simulink model "TiltCopter_TOSTO_v2"  (R2015a)
settings: Solver=ode45  StartTime=0.0  StopTime=10  RelTol=1e-3
values from neighbouring files (symbols this model uses):
  Fx = 0    [Main_tiltCopter_TOSTO.m]    (also in Main_tiltCopter_TOSTO_v2.m)
  Fy = 0    [Main_tiltCopter_TOSTO.m]    (also in Main_tiltCopter_TOSTO_v2.m = 0.2)
  U = [-1; 0; 0; 0]    [Main_tiltCopter_TOSTO.m]    (also in Main_tiltCopter_TOSTO_v2.m = [-1; 0; 0;0])
undefined symbols (not defined in the file or in its folder): b, B0, B1, B2, B3, degtorad, dLMN, g, I_Pi, In, InInv, KaD, KaI, KaN, KaP, Kba, Kbp, Kbq, Kbr, Kdp, Kdq, Kdr, Kip, Kiq, Kir, KPD, KPI, KPP, Kpp, Kpq, Kpr, Kq, KRD, KRI, KRP, Kt, m, m_servo, Mb, MbInv, N, omega_hover, pitchMax, q_servo, rollMax, satp, satq, satr, ServoMotor_Gain, tau, x1, yawRateMax
libraries: aerolibutil x10, simulink x6
(part 1 of 2)
settings Model: PauseTimes=2  Creator=Claudio  LastModifiedBy=Claudio

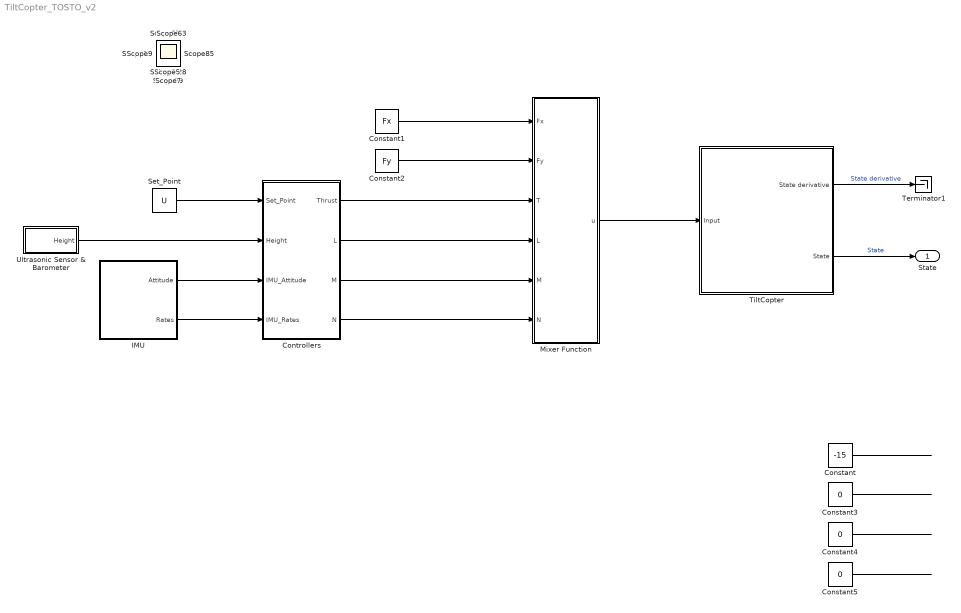
== system TiltCopter_TOSTO_v2 ==
  Constant : Constant  Value=-15
  Constant1 : Constant  Value=Fx
  Constant2 : Constant  Value=Fy
  Constant3 : Constant  Value=0
  Constant4 : Constant  Value=0
  Constant5 : Constant  Value=0
  Controllers : Subsystem
  IMU : Subsystem
  Mixer Function : Subsystem
  Set_Point : Constant  Value=U
  Terminator1 : Terminator
  TiltCopter : Subsystem
      mask Display:
      | % image(imread(''))
      | port_label('input',1,'u')
      | port_label('output',1,'Xdot')
      | port_label('output',2,'X')
  Ultrasonic Sensor & Barometer : Subsystem
  State : Outport
  Scope{,1..29} (30 alike) : Scope
      Scope settings: SaveName=ScopeData2
      Scope1 settings: SaveName=ScopeData3
      Scope10 settings: SaveName=ScopeData14
      Scope11 settings: SaveName=ScopeData15
      Scope12 settings: SaveName=ScopeData16
      Scope13 settings: SaveName=ScopeData17
      Scope14 settings: SaveName=ScopeData18
      Scope15 settings: SaveName=ScopeData19
      Scope16 settings: SaveName=ScopeData20
      Scope17 settings: SaveName=ScopeData21
      Scope18 settings: SaveName=ScopeData22
      Scope19 settings: SaveName=ScopeData23
      Scope2 settings: SaveName=ScopeData4
      Scope20 settings: SaveName=ScopeData24
      Scope21 settings: SaveName=ScopeData25
      Scope22 settings: SaveName=ScopeData26
      Scope23 settings: SaveName=ScopeData27
      Scope24 settings: SaveName=ScopeData28
      Scope25 settings: SaveName=ScopeData31
      Scope26 settings: SaveName=ScopeData30
      Scope27 settings: ShowLegends=on  SaveName=ScopeData32
      Scope28 settings: SaveName=ScopeData33
      Scope29 settings: SaveName=ScopeData34
      Scope3 settings: SaveName=ScopeData5
      Scope4 settings: SaveName=ScopeData8
      Scope5 settings: TimeRange=20  SaveName=ScopeData9
      Scope6 settings: SaveName=ScopeData10
      Scope7 settings: SaveName=ScopeData11
      Scope8 settings: SaveName=ScopeData12
      Scope9 settings: SaveName=ScopeData13
  wires:
  TiltCopter/2(State) -> State/1  "State"
  TiltCopter/1(State derivative) -> Terminator1/1  "State derivative"
  Constant1/1 -> Mixer Function/1(Fx)
  Constant2/1 -> Mixer Function/2(Fy)
  Mixer Function/1(u) -> TiltCopter/1(Input)
  Set_Point/1 -> Controllers/1(Set_Point)
  IMU/1(Attitude) -> Controllers/3(IMU_Attitude)
  IMU/2(Rates) -> Controllers/4(IMU_Rates)
  Ultrasonic Sensor & Barometer/1(Height) -> Controllers/2(Height)
  Constant/1 -> ?
  Constant5/1 -> ?
  Constant4/1 -> ?
  Constant3/1 -> ?
  Controllers/1(Thrust) -> Mixer Function/3(T)
  Controllers/2(L) -> Mixer Function/4(L)
  Controllers/3(M) -> Mixer Function/5(M)
  Controllers/4(N) -> Mixer Function/6(N)

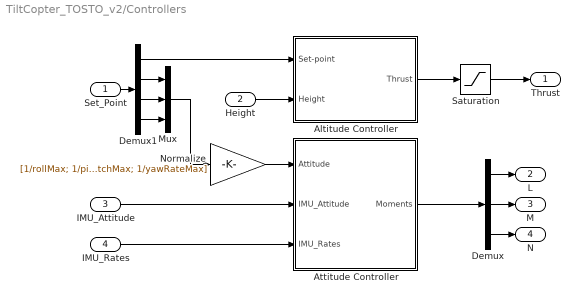
== system TiltCopter_TOSTO_v2/Controllers ==
  Set_Point : Inport
  Height : Inport  Port=2
  IMU_Attitude : Inport  Port=3
  IMU_Rates : Inport  Port=4
  Altitude Controller : Subsystem
  Attitude Controller : Subsystem
  Demux : Demux  Outputs=3
  Demux1 : Demux
  Mux : Mux  Inputs=3
  Normalize : Gain  Gain=[1/rollMax; 1/pitchMax; 1/yawRateMax]
  Saturation : Saturate  UpperLimit=0  LowerLimit=-80
  Thrust : Outport
  L : Outport  Port=2
  M : Outport  Port=3
  N : Outport  Port=4
  wires:
  IMU_Rates/1 -> Attitude Controller/3(IMU_Rates)
  Demux/1 -> L/1
  Demux/2 -> M/1
  Demux/3 -> N/1
  Set_Point/1 -> Demux1/1
  Demux1/3 -> Mux/2
  Demux1/4 -> Mux/3
  IMU_Attitude/1 -> Attitude Controller/2(IMU_Attitude)
  Mux/1 -> Normalize/1
  Normalize/1 -> Attitude Controller/1(Attitude)
  Demux1/1 -> Altitude Controller/1(Set-point)
  Height/1 -> Altitude Controller/2(Height)
  Altitude Controller/1(Thrust) -> Saturation/1
  Saturation/1 -> Thrust/1
  Attitude Controller/1(Moments) -> Demux/1
  Demux1/2 -> Mux/1

== system TiltCopter_TOSTO_v2/IMU ==
  Attitude : Outport
  Rates : Outport  Port=2
  wires:
  [Omega_b] -> Rates/1
  [Alpha_e] -> Attitude/1

== system TiltCopter_TOSTO_v2/Mixer Function ==
  Fx : Inport
  Fy : Inport  Port=2
  T : Inport  Port=3
  L : Inport  Port=4
  M : Inport  Port=5
  N : Inport  Port=6
  Mux1 : Mux
  Mux2 : Mux  Inputs=5
  NONLINEAR mixer : Subsystem
  To Workspace : ToWorkspace  VariableName=Uscita_quad  SaveFormat=Timeseries  SampleTime=-1
  u : Outport
  wires:
  Mux2/1 -> To Workspace/1, u/1
  Fy/1 -> NONLINEAR mixer/2(Fy)
  Fx/1 -> NONLINEAR mixer/1(Fx)
  T/1 -> NONLINEAR mixer/3(T)
  L/1 -> NONLINEAR mixer/4(L)
  N/1 -> NONLINEAR mixer/6(N)
  M/1 -> NONLINEAR mixer/5(M)
  Mux1/1 -> Mux2/5
  NONLINEAR mixer/5(Pulse 1 [ms]) -> Mux1/1
  NONLINEAR mixer/6(Pulse 2 [ms]) -> Mux1/2
  NONLINEAR mixer/7(Pulse 3 [ms]) -> Mux1/3
  NONLINEAR mixer/8(Pulse 4 [ms]) -> Mux1/4
  NONLINEAR mixer/4(Th4 [%]) -> Mux2/4
  NONLINEAR mixer/3(Th3 [%]) -> Mux2/3
  NONLINEAR mixer/2(Th2 [%]) -> Mux2/2
  NONLINEAR mixer/1(Th1 [%]) -> Mux2/1

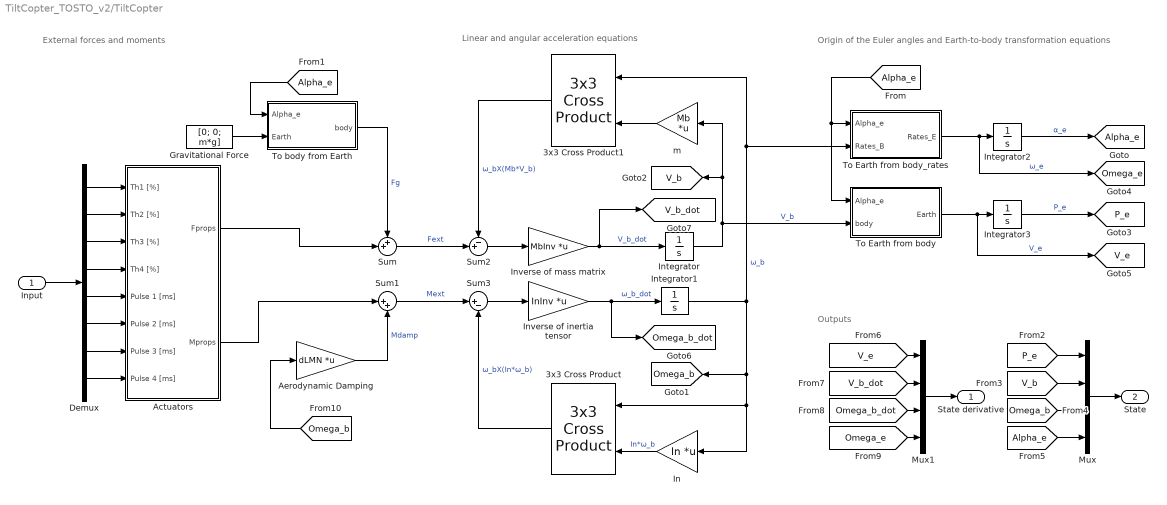
== system TiltCopter_TOSTO_v2/TiltCopter ==
  note: External forces and moments
  note: Outputs
  note: Origin of the Euler angles and Earth-to-body transformation equations
  note: Linear and angular acceleration equations
  Input : Inport
  3x3 Cross Product : aerolibutil/3x3 Cross Product
  3x3 Cross Product1 : aerolibutil/3x3 Cross Product
  Actuators : Subsystem
  Aerodynamic Damping : Gain  Gain=dLMN  Multiplication=Matrix(K*u)
  Demux : Demux  Outputs=8
  Gravitational Force : Constant  Value=[0; 0; m*g]
  In : Gain  Gain=In  Multiplication=Matrix(K*u)
  Integrator : Integrator  InitialCondition=[0; 0; 0]  UpperSaturationLimit=20
  Integrator1 : Integrator  InitialCondition=[0; 0; 0]
  Integrator2 : Integrator  InitialCondition=[0; 0; 0]
  Integrator3 : Integrator  InitialCondition=[0; 0; 0]
  Inverse of inertia tensor : Gain  Gain=InInv  Multiplication=Matrix(K*u)
  Inverse of mass matrix : Gain  Gain=MbInv  Multiplication=Matrix(K*u)
  Mux : Mux
  Mux1 : Mux
  Sum : Sum  Inputs=++|
  Sum1 : Sum  Inputs=|++
  Sum2 : Sum  Inputs=-+|
  Sum3 : Sum  Inputs=|+-
  To Earth from body : MATLAB Function  TreatAsAtomicUnit=on
  To Earth from body_rates : MATLAB Function  TreatAsAtomicUnit=on
  To body from Earth : MATLAB Function  TreatAsAtomicUnit=on
  m : Gain  Gain=Mb  Multiplication=Matrix(K*u)
  State derivative : Outport
  State : Outport  Port=2
  tag scope: Alpha_e=global, Omega_b=global, Omega_b_dot=global, Omega_e=global, P_e=global, V_b=global, V_b_dot=global, V_e=global
  wires:
  To Earth from body_rates/1(Rates_E) -> Integrator2/1, [Omega_e]  "ω_e"
  [P_e] -> Mux/1
  3x3 Cross Product/1 -> Sum3/2  "ω_bX(In*ω_b)"
  [V_b_dot] -> Mux1/2
  Mux/1 -> State/1
  Mux1/1 -> State derivative/1
  [V_b] -> Mux/2
  [Alpha_e] -> Mux/4
  [Omega_b] -> Mux/3
  Demux/4 -> Actuators/4(Th4 [%])
  [Omega_e] -> Mux1/4
  [Omega_b_dot] -> Mux1/3
  [V_e] -> Mux1/1
  Demux/3 -> Actuators/3(Th3 [%])
  Inverse of mass matrix/1 -> Integrator/1, [V_b_dot]  "V_b_dot"
  Integrator/1 -> To Earth from body/2(body), m/1, [V_b]  "V_b"
  [Alpha_e] -> To Earth from body/1(Alpha_e), To Earth from body_rates/1(Alpha_e)
  Integrator1/1 -> To Earth from body_rates/2(Rates_B), 3x3 Cross Product1/1, 3x3 Cross Product/1, In/1, [Omega_b]  "ω_b"
  Sum3/1 -> Inverse of inertia tensor/1
  Sum2/1 -> Inverse of mass matrix/1
  m/1 -> 3x3 Cross Product1/2
  Sum/1 -> Sum2/2  "Fext"
  Sum1/1 -> Sum3/1  "Mext"
  Demux/1 -> Actuators/1(Th1 [%])
  Demux/2 -> Actuators/2(Th2 [%])
  Inverse of inertia tensor/1 -> Integrator1/1, [Omega_b_dot]  "ω_b_dot"
  3x3 Cross Product1/1 -> Sum2/1  "ω_bX(Mb*V_b)"
  Integrator2/1 -> [Alpha_e]  "α_e"
  Aerodynamic Damping/1 -> Sum1/2  "Mdamp"
  Integrator3/1 -> [P_e]  "P_e"
  In/1 -> 3x3 Cross Product/2  "In*ω_b"
  [Omega_b] -> Aerodynamic Damping/1
  To Earth from body/1(Earth) -> [V_e], Integrator3/1  "V_e"
  To body from Earth/1(body) -> Sum/1  "Fg"
  Gravitational Force/1 -> To body from Earth/2(Earth)
  [Alpha_e] -> To body from Earth/1(Alpha_e)
  Input/1 -> Demux/1
  Demux/5 -> Actuators/5(Pulse 1 [ms])
  Demux/6 -> Actuators/6(Pulse 2 [ms])
  Demux/7 -> Actuators/7(Pulse 3 [ms])
  Demux/8 -> Actuators/8(Pulse 4 [ms])
  Actuators/1(Fprops) -> Sum/2
  Actuators/2(Mprops) -> Sum1/1

== system TiltCopter_TOSTO_v2/Ultrasonic Sensor & Barometer ==
  Bias_u : Bias
  Demux : Demux  Outputs=3
  Sum : Sum  Inputs=|++
  Terminator1 : Terminator
  Terminator2 : Terminator
  White Noise_u : RandomNumber  DisableCoverage=on  Variance=0*0.00001  SampleTime=0.01
  Height : Outport
  wires:
  Sum/1 -> Height/1
  Demux/2 -> Terminator1/1  "E"
  [P_e] -> Demux/1
  Bias_u/1 -> Sum/1
  White Noise_u/1 -> Sum/2
  Demux/3 -> Bias_u/1  "D"
  Demux/1 -> Terminator2/1  "N"

== system TiltCopter_TOSTO_v2/Controllers/Altitude Controller ==
  Set-point : Inport
  Height : Inport  Port=2
  Constant : Constant  Value=m*g
  Normalize : Gain
  PD Controller : simulink/Continuous/PID Controller  Controller=PID  TimeDomain=Continuous-time  SampleTime=-1  IntegratorMethod=Forward Euler  FilterMethod=Trapezoidal  Form=Parallel  UseFilter=on  ControllerParametersSource=internal  P=KaP  I=KaI  D=KaD  N=KaN  InitialConditionSource=internal  InitialConditionForIntegrator=0  InitialConditionForFilter=0  ExternalReset=none  LimitOutput=on  UpperSaturationLimit=10  LowerSaturationLimit=-10  LinearizeAsGain=on  AntiWindupMode=back-calculation  Kb=Kba  TrackingMode=off  Kt=1  PParamMin=[]  PParamMax=[]  IParamMin=[]  IParamMax=[]  DParamMin=[]  DParamMax=[]  NParamMin=[]  NParamMax=[]  KbParamMin=[]  KbParamMax=[]  KtParamMin=[]  KtParamMax=[]  POutMin=[]  POutMax=[]  IOutMin=[]  IOutMax=[]  DOutMin=[]  DOutMax=[]  NOutMin=[]  NOutMax=[]  KbOutMin=[]  KbOutMax=[]  KtOutMin=[]  KtOutMax=[]  IntegratorOutMin=[]  IntegratorOutMax=[]  FilterOutMin=[]  FilterOutMax=[]  SumOutMin=[]  SumOutMax=[]  SumI1OutMin=[]  SumI1OutMax=[]  SumI2OutMin=[]  SumI2OutMax=[]  SumI3OutMin=[]  SumI3OutMax=[]  SumDOutMin=[]  SumDOutMax=[]  SaturationOutMin=[]  SaturationOutMax=[]  IntegratorContinuousStateAttributes=''  IntegratorStateMustResolveToSignalObject=off  IntegratorRTWStateStorageClass=Auto  FilterContinuousStateAttributes=''  FilterStateMustResolveToSignalObject=off  FilterRTWStateStorageClass=Auto  DifferentiatorICPrevScaledInput=0  DifferentiatorOutMin=[]  DifferentiatorOutMax=[]
  Sum1 : Sum  Inputs=-+|
  Sum2 : Sum  Inputs=|+-
  Thrust : Outport
  wires:
  Sum2/1 -> PD Controller/1
  Height/1 -> Sum2/2
  Sum1/1 -> Thrust/1
  Constant/1 -> Sum1/1
  Set-point/1 -> Sum2/1
  PD Controller/1 -> Normalize/1
  Normalize/1 -> Sum1/2

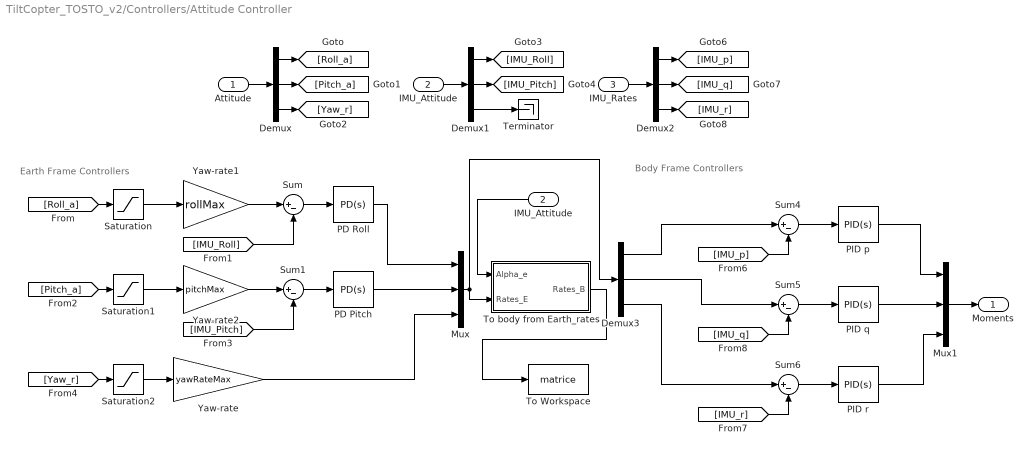
== system TiltCopter_TOSTO_v2/Controllers/Attitude Controller ==
  note: Body Frame Controllers
  note: Earth Frame Controllers
  Attitude : Inport
  IMU_Attitude : Inport  Port=2
  IMU_Rates : Inport  Port=3
  Demux{,1..3} (4 alike) : Demux  Outputs=3
  "IMU_Attitude " : InportShadow  Port=2
  Mux : Mux  Inputs=3
  Mux1 : Mux  Inputs=3
  PD Pitch : simulink/Continuous/PID Controller  Controller=PD  TimeDomain=Continuous-time  SampleTime=-1  IntegratorMethod=Forward Euler  FilterMethod=Forward Euler  Form=Parallel  UseFilter=on  ControllerParametersSource=internal  P=KPP  I=KPI  D=KPD  N=N  InitialConditionSource=internal  InitialConditionForIntegrator=0  InitialConditionForFilter=0  ExternalReset=none  LimitOutput=off  UpperSaturationLimit=inf  LowerSaturationLimit=-inf  LinearizeAsGain=on  AntiWindupMode=none  Kb=1  TrackingMode=off  Kt=1  PParamMin=[]  PParamMax=[]  IParamMin=[]  IParamMax=[]  DParamMin=[]  DParamMax=[]  NParamMin=[]  NParamMax=[]  KbParamMin=[]  KbParamMax=[]  KtParamMin=[]  KtParamMax=[]  POutMin=[]  POutMax=[]  IOutMin=[]  IOutMax=[]  DOutMin=[]  DOutMax=[]  NOutMin=[]  NOutMax=[]  KbOutMin=[]  KbOutMax=[]  KtOutMin=[]  KtOutMax=[]  IntegratorOutMin=[]  IntegratorOutMax=[]  FilterOutMin=[]  FilterOutMax=[]  SumOutMin=[]  SumOutMax=[]  SumI1OutMin=[]  SumI1OutMax=[]  SumI2OutMin=[]  SumI2OutMax=[]  SumI3OutMin=[]  SumI3OutMax=[]  SumDOutMin=[]  SumDOutMax=[]  SaturationOutMin=[]  SaturationOutMax=[]  IntegratorContinuousStateAttributes=''  IntegratorStateMustResolveToSignalObject=off  IntegratorRTWStateStorageClass=Auto  FilterContinuousStateAttributes=''  FilterStateMustResolveToSignalObject=off  FilterRTWStateStorageClass=Auto  DifferentiatorICPrevScaledInput=0  DifferentiatorOutMin=[]  DifferentiatorOutMax=[]
  PD Roll : simulink/Continuous/PID Controller  Controller=PD  TimeDomain=Continuous-time  SampleTime=-1  IntegratorMethod=Forward Euler  FilterMethod=Forward Euler  Form=Parallel  UseFilter=on  ControllerParametersSource=internal  P=KRP  I=KRI  D=KRD  N=N  InitialConditionSource=internal  InitialConditionForIntegrator=0  InitialConditionForFilter=0  ExternalReset=none  LimitOutput=off  UpperSaturationLimit=inf  LowerSaturationLimit=-inf  LinearizeAsGain=on  AntiWindupMode=none  Kb=1  TrackingMode=off  Kt=1  PParamMin=[]  PParamMax=[]  IParamMin=[]  IParamMax=[]  DParamMin=[]  DParamMax=[]  NParamMin=[]  NParamMax=[]  KbParamMin=[]  KbParamMax=[]  KtParamMin=[]  KtParamMax=[]  POutMin=[]  POutMax=[]  IOutMin=[]  IOutMax=[]  DOutMin=[]  DOutMax=[]  NOutMin=[]  NOutMax=[]  KbOutMin=[]  KbOutMax=[]  KtOutMin=[]  KtOutMax=[]  IntegratorOutMin=[]  IntegratorOutMax=[]  FilterOutMin=[]  FilterOutMax=[]  SumOutMin=[]  SumOutMax=[]  SumI1OutMin=[]  SumI1OutMax=[]  SumI2OutMin=[]  SumI2OutMax=[]  SumI3OutMin=[]  SumI3OutMax=[]  SumDOutMin=[]  SumDOutMax=[]  SaturationOutMin=[]  SaturationOutMax=[]  IntegratorContinuousStateAttributes=''  IntegratorStateMustResolveToSignalObject=off  IntegratorRTWStateStorageClass=Auto  FilterContinuousStateAttributes=''  FilterStateMustResolveToSignalObject=off  FilterRTWStateStorageClass=Auto  DifferentiatorICPrevScaledInput=0  DifferentiatorOutMin=[]  DifferentiatorOutMax=[]
  PID p : simulink/Continuous/PID Controller  Controller=PID  TimeDomain=Continuous-time  SampleTime=-1  IntegratorMethod=Forward Euler  FilterMethod=Forward Euler  Form=Parallel  UseFilter=on  ControllerParametersSource=internal  P=Kpp  I=Kip  D=Kdp  N=N  InitialConditionSource=internal  InitialConditionForIntegrator=0  InitialConditionForFilter=0  ExternalReset=none  LimitOutput=on  UpperSaturationLimit=satp  LowerSaturationLimit=-satp  LinearizeAsGain=on  AntiWindupMode=back-calculation  Kb=Kbp  TrackingMode=off  Kt=1  PParamMin=[]  PParamMax=[]  IParamMin=[]  IParamMax=[]  DParamMin=[]  DParamMax=[]  NParamMin=[]  NParamMax=[]  KbParamMin=[]  KbParamMax=[]  KtParamMin=[]  KtParamMax=[]  POutMin=[]  POutMax=[]  IOutMin=[]  IOutMax=[]  DOutMin=[]  DOutMax=[]  NOutMin=[]  NOutMax=[]  KbOutMin=[]  KbOutMax=[]  KtOutMin=[]  KtOutMax=[]  IntegratorOutMin=[]  IntegratorOutMax=[]  FilterOutMin=[]  FilterOutMax=[]  SumOutMin=[]  SumOutMax=[]  SumI1OutMin=[]  SumI1OutMax=[]  SumI2OutMin=[]  SumI2OutMax=[]  SumI3OutMin=[]  SumI3OutMax=[]  SumDOutMin=[]  SumDOutMax=[]  SaturationOutMin=[]  SaturationOutMax=[]  IntegratorContinuousStateAttributes=''  IntegratorStateMustResolveToSignalObject=off  IntegratorRTWStateStorageClass=Auto  FilterContinuousStateAttributes=''  FilterStateMustResolveToSignalObject=off  FilterRTWStateStorageClass=Auto  DifferentiatorICPrevScaledInput=0  DifferentiatorOutMin=[]  DifferentiatorOutMax=[]
  PID q : simulink/Continuous/PID Controller  Controller=PID  TimeDomain=Continuous-time  SampleTime=-1  IntegratorMethod=Forward Euler  FilterMethod=Forward Euler  Form=Parallel  UseFilter=on  ControllerParametersSource=internal  P=Kpq  I=Kiq  D=Kdq  N=N  InitialConditionSource=internal  InitialConditionForIntegrator=0  InitialConditionForFilter=0  ExternalReset=none  LimitOutput=on  UpperSaturationLimit=satq  LowerSaturationLimit=-satq  LinearizeAsGain=on  AntiWindupMode=back-calculation  Kb=Kbq  TrackingMode=off  Kt=1  PParamMin=[]  PParamMax=[]  IParamMin=[]  IParamMax=[]  DParamMin=[]  DParamMax=[]  NParamMin=[]  NParamMax=[]  KbParamMin=[]  KbParamMax=[]  KtParamMin=[]  KtParamMax=[]  POutMin=[]  POutMax=[]  IOutMin=[]  IOutMax=[]  DOutMin=[]  DOutMax=[]  NOutMin=[]  NOutMax=[]  KbOutMin=[]  KbOutMax=[]  KtOutMin=[]  KtOutMax=[]  IntegratorOutMin=[]  IntegratorOutMax=[]  FilterOutMin=[]  FilterOutMax=[]  SumOutMin=[]  SumOutMax=[]  SumI1OutMin=[]  SumI1OutMax=[]  SumI2OutMin=[]  SumI2OutMax=[]  SumI3OutMin=[]  SumI3OutMax=[]  SumDOutMin=[]  SumDOutMax=[]  SaturationOutMin=[]  SaturationOutMax=[]  IntegratorContinuousStateAttributes=''  IntegratorStateMustResolveToSignalObject=off  IntegratorRTWStateStorageClass=Auto  FilterContinuousStateAttributes=''  FilterStateMustResolveToSignalObject=off  FilterRTWStateStorageClass=Auto  DifferentiatorICPrevScaledInput=0  DifferentiatorOutMin=[]  DifferentiatorOutMax=[]
  PID r : simulink/Continuous/PID Controller  Controller=PID  TimeDomain=Continuous-time  SampleTime=-1  IntegratorMethod=Forward Euler  FilterMethod=Forward Euler  Form=Parallel  UseFilter=on  ControllerParametersSource=internal  P=Kpr  I=Kir  D=Kdr  N=N  InitialConditionSource=internal  InitialConditionForIntegrator=0  InitialConditionForFilter=0  ExternalReset=none  LimitOutput=on  UpperSaturationLimit=satr  LowerSaturationLimit=-satr  LinearizeAsGain=on  AntiWindupMode=back-calculation  Kb=Kbr  TrackingMode=off  Kt=1  PParamMin=[]  PParamMax=[]  IParamMin=[]  IParamMax=[]  DParamMin=[]  DParamMax=[]  NParamMin=[]  NParamMax=[]  KbParamMin=[]  KbParamMax=[]  KtParamMin=[]  KtParamMax=[]  POutMin=[]  POutMax=[]  IOutMin=[]  IOutMax=[]  DOutMin=[]  DOutMax=[]  NOutMin=[]  NOutMax=[]  KbOutMin=[]  KbOutMax=[]  KtOutMin=[]  KtOutMax=[]  IntegratorOutMin=[]  IntegratorOutMax=[]  FilterOutMin=[]  FilterOutMax=[]  SumOutMin=[]  SumOutMax=[]  SumI1OutMin=[]  SumI1OutMax=[]  SumI2OutMin=[]  SumI2OutMax=[]  SumI3OutMin=[]  SumI3OutMax=[]  SumDOutMin=[]  SumDOutMax=[]  SaturationOutMin=[]  SaturationOutMax=[]  IntegratorContinuousStateAttributes=''  IntegratorStateMustResolveToSignalObject=off  IntegratorRTWStateStorageClass=Auto  FilterContinuousStateAttributes=''  FilterStateMustResolveToSignalObject=off  FilterRTWStateStorageClass=Auto  DifferentiatorICPrevScaledInput=0  DifferentiatorOutMin=[]  DifferentiatorOutMax=[]
  Saturation : Saturate  UpperLimit=1  LowerLimit=-1
  Saturation1 : Saturate  UpperLimit=1  LowerLimit=-1
  Saturation2 : Saturate  UpperLimit=1  LowerLimit=-1
  Sum{,1,4..6} (5 alike) : Sum  Inputs=|+-
  Terminator : Terminator
  To Workspace : ToWorkspace  VariableName=matrice  SaveFormat=Timeseries  SampleTime=-1
  To body from Earth_rates : MATLAB Function  TreatAsAtomicUnit=on
  Yaw-rate : Gain  Gain=yawRateMax
  Yaw-rate1 : Gain  Gain=rollMax
  Yaw-rate2 : Gain  Gain=pitchMax
  Moments : Outport
  wires:
  Sum4/1 -> PID p/1
  IMU_Attitude/1 -> Demux1/1
  Attitude/1 -> Demux/1
  Demux/3 -> [Yaw_r]
  IMU_Rates/1 -> Demux2/1
  [IMU_Pitch] -> Sum1/2
  [Pitch_a] -> Saturation1/1
  [IMU_Roll] -> Sum/2
  [Roll_a] -> Saturation/1
  Mux1/1 -> Moments/1
  PD Roll/1 -> Mux/1
  [Yaw_r] -> Saturation2/1
  PD Pitch/1 -> Mux/2
  Sum5/1 -> PID q/1
  PID r/1 -> Mux1/3
  PID p/1 -> Mux1/1
  Sum6/1 -> PID r/1
  PID q/1 -> Mux1/2
  Demux/2 -> [Pitch_a]
  Demux2/3 -> [IMU_r]
  Demux1/1 -> [IMU_Roll]
  Demux/1 -> [Roll_a]
  Demux2/1 -> [IMU_p]
  Demux1/3 -> Terminator/1
  Demux2/2 -> [IMU_q]
  Demux1/2 -> [IMU_Pitch]
  Sum/1 -> PD Roll/1
  Sum1/1 -> PD Pitch/1
  Saturation1/1 -> Yaw-rate2/1
  Yaw-rate1/1 -> Sum/1
  Yaw-rate2/1 -> Sum1/1
  Demux3/1 -> Sum4/1
  [IMU_p] -> Sum4/2
  Demux3/2 -> Sum5/1
  Demux3/3 -> Sum6/1
  [IMU_q] -> Sum5/2
  [IMU_r] -> Sum6/2
  Yaw-rate/1 -> Mux/3
  Saturation/1 -> Yaw-rate1/1
  Saturation2/1 -> Yaw-rate/1
  "IMU_Attitude "/1 -> To body from Earth_rates/1(Alpha_e)
  To body from Earth_rates/1(Rates_B) -> To Workspace/1
  Mux/1 -> Demux3/1, To body from Earth_rates/2(Rates_E)

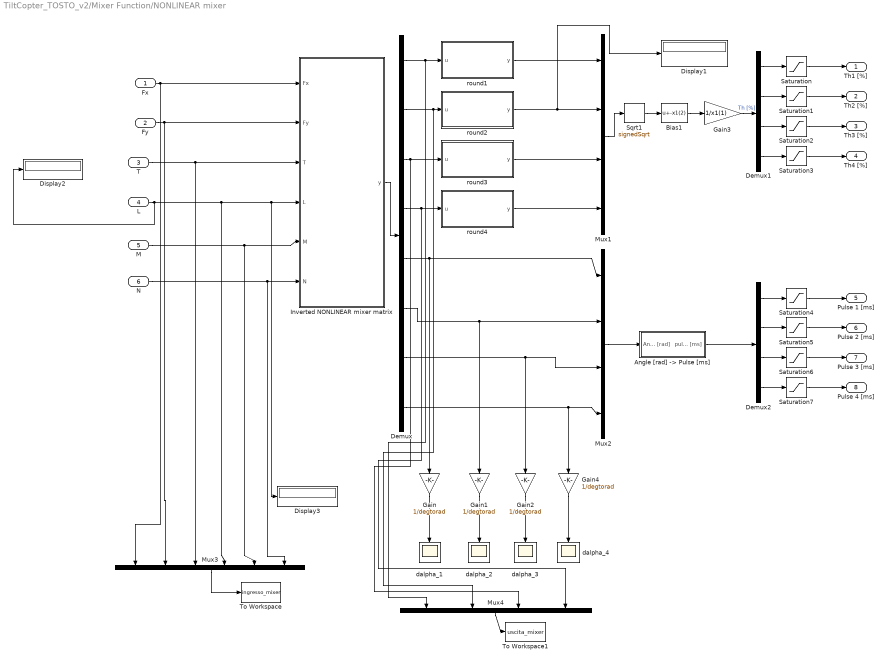
== system TiltCopter_TOSTO_v2/Mixer Function/NONLINEAR mixer ==
  Fx : Inport
  Fy : Inport  Port=2
  T : Inport  Port=3
  L : Inport  Port=4
  M : Inport  Port=5
  N : Inport  Port=6
  "Angle [rad] -> Pulse [ms]" : Subsystem
  Bias1 : Bias  Bias=-x1(2)
  Demux : Demux  Outputs=8
  Demux1 : Demux
  Demux2 : Demux
  Display1 : Display
  Display2 : Display
  Display3 : Display
  Gain{,1..2,4} (4 alike) : Gain  Gain=1/degtorad
  Gain3 : Gain  Gain=1/x1(1)
  Inverted NONLINEAR mixer matrix : MATLAB Function  TreatAsAtomicUnit=on
  Mux1 : Mux
  Mux2 : Mux
  Mux3 : Mux  Inputs=6
  Mux4 : Mux
  Saturation{,1..3} (4 alike) : Saturate  UpperLimit=100  LowerLimit=0
  Saturation{4..7} (4 alike) : Saturate  UpperLimit=2000  LowerLimit=1000
  Sqrt1 : Sqrt  Operator=signedSqrt  SaturateOnIntegerOverflow=on
  To Workspace : ToWorkspace  VariableName=ingresso_mixer  SaveFormat=Structure With Time  SampleTime=-1
  To Workspace1 : ToWorkspace  VariableName=uscita_mixer  SaveFormat=Structure With Time  SampleTime=-1
  dalpha_{1..4} (4 alike) : Scope
      dalpha_3 settings: SaveName=ScopeData6
      dalpha_4 settings: SaveName=ScopeData7
  round1 : MATLAB Function  TreatAsAtomicUnit=on
  round2 : MATLAB Function  TreatAsAtomicUnit=on
  round3 : MATLAB Function  TreatAsAtomicUnit=on
  round4 : MATLAB Function  TreatAsAtomicUnit=on
  Th1 [%] : Outport
  Th2 [%] : Outport  Port=2
  Th3 [%] : Outport  Port=3
  Th4 [%] : Outport  Port=4
  Pulse 1 [ms] : Outport  Port=5
  Pulse 2 [ms] : Outport  Port=6
  Pulse 3 [ms] : Outport  Port=7
  Pulse 4 [ms] : Outport  Port=8
  wires:
  round1/1(y) -> Mux1/1
  Saturation6/1 -> Pulse 3 [ms]/1
  Demux2/1 -> Saturation4/1
  Demux2/3 -> Saturation6/1
  Demux/4 -> Mux4/4, round4/1(u)
  Saturation2/1 -> Th3 [%]/1
  Demux1/2 -> Saturation1/1
  Demux1/1 -> Saturation/1
  Demux1/3 -> Saturation2/1
  Demux1/4 -> Saturation3/1
  Saturation1/1 -> Th2 [%]/1
  Gain3/1 -> Demux1/1  "Th [%]"
  Sqrt1/1 -> Bias1/1
  Mux1/1 -> Sqrt1/1
  Demux/1 -> Mux4/1, round1/1(u)
  Bias1/1 -> Gain3/1
  Saturation3/1 -> Th4 [%]/1
  Saturation/1 -> Th1 [%]/1
  Demux2/2 -> Saturation5/1
  round2/1(y) -> Display1/1, Mux1/2
  round4/1(y) -> Mux1/4
  Demux/7 -> Gain2/1, Mux2/3
  Demux/5 -> Gain/1, Mux2/1
  Demux/6 -> Mux2/2, Gain1/1
  Mux2/1 -> "Angle [rad] -> Pulse [ms]"/1(Angle [rad])
  Demux2/4 -> Saturation7/1
  Demux/3 -> round3/1(u), Mux4/3
  Demux/8 -> Mux2/4, Gain4/1
  "Angle [rad] -> Pulse [ms]"/1(pulse [ms]) -> Demux2/1
  Saturation4/1 -> Pulse 1 [ms]/1
  Saturation5/1 -> Pulse 2 [ms]/1
  Saturation7/1 -> Pulse 4 [ms]/1
  Gain1/1 -> dalpha_2/1
  Gain/1 -> dalpha_1/1
  Gain2/1 -> dalpha_3/1
  Gain4/1 -> dalpha_4/1
  round3/1(y) -> Mux1/3
  Inverted NONLINEAR mixer matrix/1(y) -> Demux/1
  Demux/2 -> Mux4/2, round2/1(u)
  Fx/1 -> Mux3/1, Inverted NONLINEAR mixer matrix/1(Fx)
  Fy/1 -> Inverted NONLINEAR mixer matrix/2(Fy), Mux3/2
  T/1 -> Inverted NONLINEAR mixer matrix/3(T), Mux3/3
  L/1 -> Mux3/4, Display3/1, Inverted NONLINEAR mixer matrix/4(L), Display2/1
  M/1 -> Mux3/5, Inverted NONLINEAR mixer matrix/5(M)
  N/1 -> Mux3/6, Inverted NONLINEAR mixer matrix/6(N)
  Mux3/1 -> To Workspace/1
  Mux4/1 -> To Workspace1/1

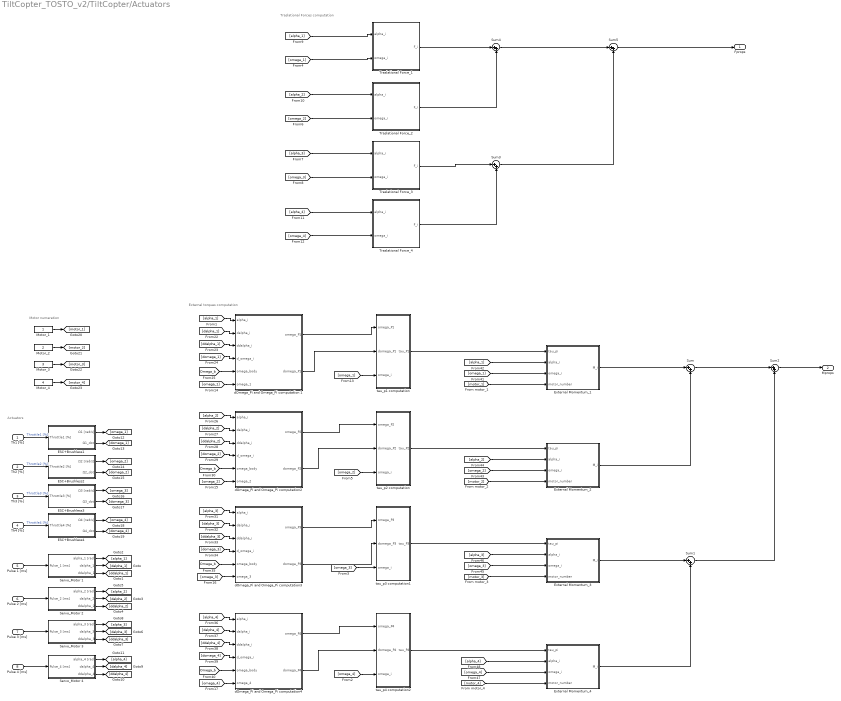
== system TiltCopter_TOSTO_v2/TiltCopter/Actuators ==
  note: Actuators
  note: Motor numeration
  note: External torques computation
  note: Traslational Forces computation
  Th1 [%] : Inport
  Th2 [%] : Inport  Port=2
  Th3 [%] : Inport  Port=3
  Th4 [%] : Inport  Port=4
  Pulse 1 [ms] : Inport  Port=5
  Pulse 2 [ms] : Inport  Port=6
  Pulse 3 [ms] : Inport  Port=7
  Pulse 4 [ms] : Inport  Port=8
  ESC+Brushless1 : Subsystem
  ESC+Brushless2 : Subsystem
  ESC+Brushless3 : Subsystem
  ESC+Brushless4 : Subsystem
  External Momentum_1 : Subsystem
  External Momentum_2 : Subsystem
  External Momentum_3 : Subsystem
  External Momentum_4 : Subsystem
  Motor_1 : Constant
  Motor_2 : Constant  Value=2
  Motor_3 : Constant  Value=3
  Motor_4 : Constant  Value=4
  Servo_Motor 1 : Subsystem
  Servo_Motor 2 : Subsystem
  Servo_Motor 3 : Subsystem
  Servo_Motor 4 : Subsystem
  Sum{,1..5} (6 alike) : Sum  Inputs=|++
  Traslational Force_1 : Subsystem
  Traslational Force_2 : Subsystem
  Traslational Force_3 : Subsystem
  Traslational Force_4 : Subsystem
  dOmega_Pi and Omega_Pi computation 1 : Subsystem
  dOmega_Pi and Omega_Pi computation2 : Subsystem
  dOmega_Pi and Omega_Pi computation3 : Subsystem
  dOmega_Pi and Omega_Pi computation4 : Subsystem
  tau_p1 computation : Subsystem
  tau_p2 computation : Subsystem
  tau_p3 computation1 : Subsystem
  tau_p4 computation2 : Subsystem
  Fprops : Outport
  Mprops : Outport  Port=2
  wires:
  Th1 [%]/1 -> ESC+Brushless1/1(Throttle1 [%])  "Throttle1 [%]"
  Th2 [%]/1 -> ESC+Brushless2/1(Throttle2 [%])  "Throttle2 [%]"
  Th4 [%]/1 -> ESC+Brushless4/1(Throttle4 [%])  "Throttle4 [%]"
  Th3 [%]/1 -> ESC+Brushless3/1(Throttle3 [%])  "Throttle3 [%]"
  Pulse 1 [ms]/1 -> Servo_Motor 1/1(Pulse_1 [ms])
  Pulse 2 [ms]/1 -> Servo_Motor 2/1(Pulse_2 [ms])
  Pulse 3 [ms]/1 -> Servo_Motor 3/1(Pulse_3 [ms])
  Pulse 4 [ms]/1 -> Servo_Motor 4/1(Pulse_4 [ms])
  Servo_Motor 1/2(dalpha_1) -> [dalpha_1]
  Servo_Motor 1/3(ddalpha_1) -> [ddalpha_1]
  Servo_Motor 3/1(alpha_3 [rad]) -> [alpha_3]
  Servo_Motor 3/3(ddalpha_3) -> [ddalpha_3]
  Servo_Motor 3/2(dalpha_3) -> [dalpha_3]
  Servo_Motor 2/3(ddalpha_2) -> [ddalpha_2]
  Servo_Motor 2/2(dalpha_2) -> [dalpha_2]
  Servo_Motor 2/1(alpha_2 [rad]) -> [alpha_2]
  Servo_Motor 1/1(alpha_1 [rad]) -> [alpha_1]
  Servo_Motor 4/1(alpha_4 [rad]) -> [alpha_4]
  Servo_Motor 4/2(dalpha_4) -> [dalpha_4]
  Servo_Motor 4/3(ddalpha_4) -> [ddalpha_4]
  ESC+Brushless1/1(Ω1 [rad/s]) -> [omega_1]
  ESC+Brushless1/2(Ω1_dot) -> [domega_1]
  ESC+Brushless2/1(Ω2 [rad/s]) -> [omega_2]
  ESC+Brushless2/2(Ω2_dot) -> [domega_2]
  ESC+Brushless3/1(Ω3 [rad/s]) -> [omega_3]
  ESC+Brushless3/2(Ω3_dot) -> [domega_3]
  ESC+Brushless4/1(Ω4 [rad/s]) -> [omega_4]
  ESC+Brushless4/2("Ω4_dot ") -> [domega_4]
  [alpha_1] -> dOmega_Pi and Omega_Pi computation 1/1(alpha_i)
  [dalpha_1] -> dOmega_Pi and Omega_Pi computation 1/2(dalpha_i)
  [ddalpha_1] -> dOmega_Pi and Omega_Pi computation 1/3(ddalpha_i)
  [domega_1] -> dOmega_Pi and Omega_Pi computation 1/4(d_omega_i)
  [Omega_b] -> dOmega_Pi and Omega_Pi computation 1/5(omega_body)
  [alpha_2] -> dOmega_Pi and Omega_Pi computation2/1(alpha_i)
  [dalpha_2] -> dOmega_Pi and Omega_Pi computation2/2(dalpha_i)
  [ddalpha_2] -> dOmega_Pi and Omega_Pi computation2/3(ddalpha_i)
  [domega_2] -> dOmega_Pi and Omega_Pi computation2/4(d_omega_i)
  [Omega_b] -> dOmega_Pi and Omega_Pi computation2/5(omega_body)
  [alpha_3] -> dOmega_Pi and Omega_Pi computation3/1(alpha_i)
  [dalpha_3] -> dOmega_Pi and Omega_Pi computation3/2(dalpha_i)
  [ddalpha_3] -> dOmega_Pi and Omega_Pi computation3/3(ddalpha_i)
  [domega_3] -> dOmega_Pi and Omega_Pi computation3/4(d_omega_i)
  [Omega_b] -> dOmega_Pi and Omega_Pi computation3/5(omega_body)
  [alpha_4] -> dOmega_Pi and Omega_Pi computation4/1(alpha_i)
  [dalpha_4] -> dOmega_Pi and Omega_Pi computation4/2(dalpha_i)
  [ddalpha_4] -> dOmega_Pi and Omega_Pi computation4/3(ddalpha_i)
  [domega_4] -> dOmega_Pi and Omega_Pi computation4/4(d_omega_i)
  [Omega_b] -> dOmega_Pi and Omega_Pi computation4/5(omega_body)
  dOmega_Pi and Omega_Pi computation 1/1(omega_P1) -> tau_p1 computation/1(omega_P1)
  dOmega_Pi and Omega_Pi computation 1/2(domega_P1) -> tau_p1 computation/2(domega_P1)
  dOmega_Pi and Omega_Pi computation2/1(omega_P2) -> tau_p2 computation/1(omega_P2)
  dOmega_Pi and Omega_Pi computation2/2(domega_P2) -> tau_p2 computation/2(domega_P2)
  dOmega_Pi and Omega_Pi computation3/1(omega_P3) -> tau_p3 computation1/1(omega_P3)
  dOmega_Pi and Omega_Pi computation3/2(domega_P3) -> tau_p3 computation1/2(domega_P3)
  dOmega_Pi and Omega_Pi computation4/1(omega_P4) -> tau_p4 computation2/1(omega_P4)
  dOmega_Pi and Omega_Pi computation4/2(domega_P4) -> tau_p4 computation2/2(domega_P4)
  tau_p1 computation/1(tau_P1) -> External Momentum_1/1(tau_pi)
  [alpha_1] -> External Momentum_1/2(alpha_i)
  [omega_1] -> External Momentum_1/3(omega_i)
  tau_p2 computation/1(tau_P2) -> External Momentum_2/1(tau_pi)
  [alpha_2] -> External Momentum_2/2(alpha_i)
  [omega_2] -> External Momentum_2/3(omega_i)
  [motor_2] -> External Momentum_2/4(motor_number)
  tau_p3 computation1/1(tau_P3) -> External Momentum_3/1(tau_pi)
  [alpha_3] -> External Momentum_3/2(alpha_i)
  [omega_3] -> External Momentum_3/3(omega_i)
  [motor_3] -> External Momentum_3/4(motor_number)
  [alpha_4] -> External Momentum_4/2(alpha_i)
  [omega_4] -> External Momentum_4/3(omega_i)
  [motor_4] -> External Momentum_4/4(motor_number)
  tau_p4 computation2/1(tau_P4) -> External Momentum_4/1(tau_pi)
  External Momentum_1/1(M_i) -> Sum/1
  External Momentum_3/1(M_i) -> Sum1/1
  External Momentum_4/1(M_i) -> Sum1/2
  Sum/1 -> Sum2/1
  Sum2/1 -> Mprops/1
  [omega_2] -> Traslational Force_2/2(omega_i)
  [alpha_1] -> Traslational Force_1/1(alpha_i)
  [omega_1] -> Traslational Force_1/2(omega_i)
  [alpha_2] -> Traslational Force_2/1(alpha_i)
  Motor_1/1 -> [motor_1]
  Motor_2/1 -> [motor_2]
  Motor_3/1 -> [motor_3]
  Motor_4/1 -> [motor_4]
  [omega_3] -> Traslational Force_3/2(omega_i)
  [alpha_3] -> Traslational Force_3/1(alpha_i)
  [omega_4] -> Traslational Force_4/2(omega_i)
  [alpha_4] -> Traslational Force_4/1(alpha_i)
  Traslational Force_3/1(F_i) -> Sum3/1
  Traslational Force_4/1(F_i) -> Sum3/2
  Traslational Force_1/1(F_i) -> Sum4/1
  Traslational Force_2/1(F_i) -> Sum4/2
  Sum4/1 -> Sum5/1
  Sum3/1 -> Sum5/2
  Sum5/1 -> Fprops/1
  [omega_4] -> tau_p4 computation2/3(omega_i)
  [omega_3] -> tau_p3 computation1/3(omega_i)
  [omega_2] -> tau_p2 computation/3(omega_i)
  [omega_1] -> tau_p1 computation/3(omega_i)
  Sum1/1 -> Sum2/2
  External Momentum_2/1(M_i) -> Sum/2
  [motor_1] -> External Momentum_1/4(motor_number)
  [omega_1] -> dOmega_Pi and Omega_Pi computation 1/6(omega_1)
  [omega_2] -> dOmega_Pi and Omega_Pi computation2/6(omega_2)
  [omega_3] -> dOmega_Pi and Omega_Pi computation3/6(omega_3)
  [omega_4] -> dOmega_Pi and Omega_Pi computation4/6(omega_4)

== system TiltCopter_TOSTO_v2/Mixer Function/NONLINEAR mixer/Angle [rad] -> Pulse [ms] ==
  Angle [rad] : Inport
  Add : Sum
  Constant : Constant  Value=q_servo
  Linear fitting gain : Gain  Gain=m_servo
  pulse [ms] : Outport
  wires:
  Angle [rad]/1 -> Linear fitting gain/1
  Constant/1 -> Add/2
  Linear fitting gain/1 -> Add/1
  Add/1 -> pulse [ms]/1

== system TiltCopter_TOSTO_v2/TiltCopter/Actuators/ESC+Brushless1 ==
  note: questo blocco è stato introdotto per avere in
      | uscita l'accelerazione e la velocità
  Throttle1 [%] : Inport
  Bias : Bias  Bias=x1(2)
  Derivative : Derivative
  Gain : Gain  Gain=x1(1)
  Transfer Fcn : TransferFcn  Denominator=[(tau) 1]
  Ω1 [rad/s] : Outport
  Ω1_dot : Outport  Port=2
  wires:
  Bias/1 -> Ω1 [rad/s]/1
  Throttle1 [%]/1 -> Transfer Fcn/1
  Transfer Fcn/1 -> Gain/1
  Gain/1 -> Bias/1, Derivative/1
  Derivative/1 -> Ω1_dot/1

== system TiltCopter_TOSTO_v2/TiltCopter/Actuators/ESC+Brushless2 ==
  Throttle2 [%] : Inport
  Bias : Bias  Bias=x1(2)
  Derivative : Derivative
  Gain : Gain  Gain=x1(1)
  Transfer Fcn : TransferFcn  Denominator=[(tau) 1]
  Ω2 [rad/s] : Outport
  Ω2_dot : Outport  Port=2
  wires:
  Bias/1 -> Ω2 [rad/s]/1
  Throttle2 [%]/1 -> Transfer Fcn/1
  Transfer Fcn/1 -> Gain/1
  Gain/1 -> Derivative/1, Bias/1
  Derivative/1 -> Ω2_dot/1

== system TiltCopter_TOSTO_v2/TiltCopter/Actuators/ESC+Brushless3 ==
  Throttle3 [%] : Inport
  Bias : Bias  Bias=x1(2)
  Derivative : Derivative
  Gain : Gain  Gain=x1(1)
  Switch : Switch  Criteria=u2 > Threshold
  Transfer Fcn : TransferFcn  Denominator=[(tau) 1]
  Ω3 [rad/s] : Outport
  Ω3_dot : Outport  Port=2
  wires:
  Gain/1 -> Bias/1
  Bias/1 -> Derivative/1, Ω3 [rad/s]/1
  Throttle3 [%]/1 -> Transfer Fcn/1
  Transfer Fcn/1 -> Gain/1
  Derivative/1 -> Ω3_dot/1

== system TiltCopter_TOSTO_v2/TiltCopter/Actuators/ESC+Brushless4 ==
  Throttle4 [%] : Inport
  Bias : Bias  Bias=x1(2)
  Derivative : Derivative
  Gain : Gain  Gain=x1(1)
  Transfer Fcn : TransferFcn  Denominator=[(tau) 1]
  Ω4 [rad/s] : Outport
  "Ω4_dot " : Outport  Port=2
  wires:
  Gain/1 -> Bias/1
  Throttle4 [%]/1 -> Transfer Fcn/1
  Transfer Fcn/1 -> Gain/1
  Derivative/1 -> "Ω4_dot "/1
  Bias/1 -> Derivative/1, Ω4 [rad/s]/1

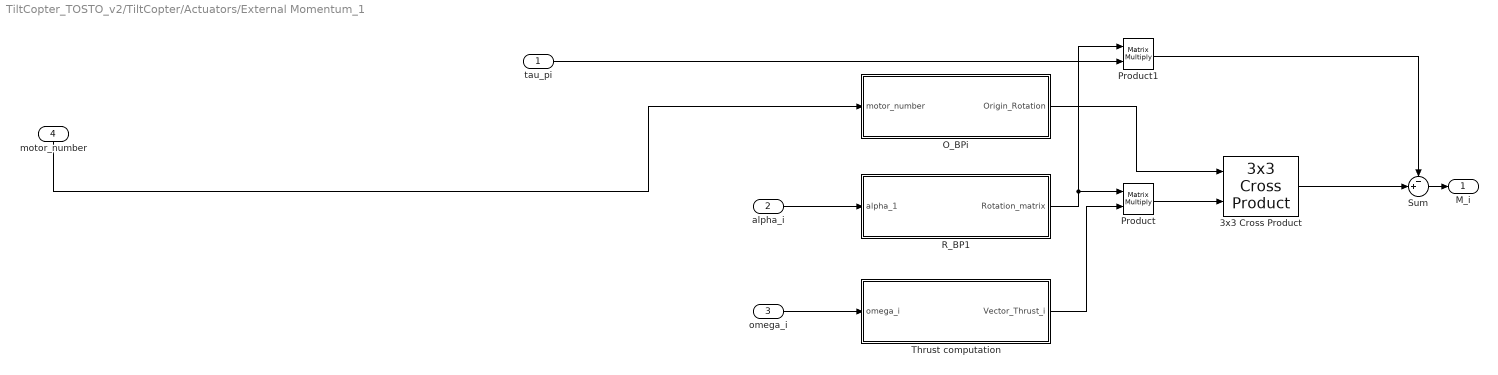
== system TiltCopter_TOSTO_v2/TiltCopter/Actuators/External Momentum_1 ==
  tau_pi : Inport
  alpha_i : Inport  Port=2
  omega_i : Inport  Port=3
  motor_number : Inport  Port=4
  3x3 Cross Product : aerolibutil/3x3 Cross Product
  O_BPi : MATLAB Function  TreatAsAtomicUnit=on
  Product : Product  Multiplication=Matrix(*)
  Product1 : Product  Multiplication=Matrix(*)
  R_BP1 : MATLAB Function  TreatAsAtomicUnit=on
  Sum : Sum  Inputs=-+|
  Thrust computation : Subsystem
  M_i : Outport
  wires:
  Sum/1 -> M_i/1
  R_BP1/1(Rotation_matrix) -> Product1/1, Product/1
  alpha_i/1 -> R_BP1/1(alpha_1)
  Product/1 -> 3x3 Cross Product/2
  tau_pi/1 -> Product1/2
  motor_number/1 -> O_BPi/1(motor_number)
  omega_i/1 -> Thrust computation/1(omega_i)
  Thrust computation/1(Vector_Thrust_i) -> Product/2
  3x3 Cross Product/1 -> Sum/2
  Product1/1 -> Sum/1
  O_BPi/1(Origin_Rotation) -> 3x3 Cross Product/1

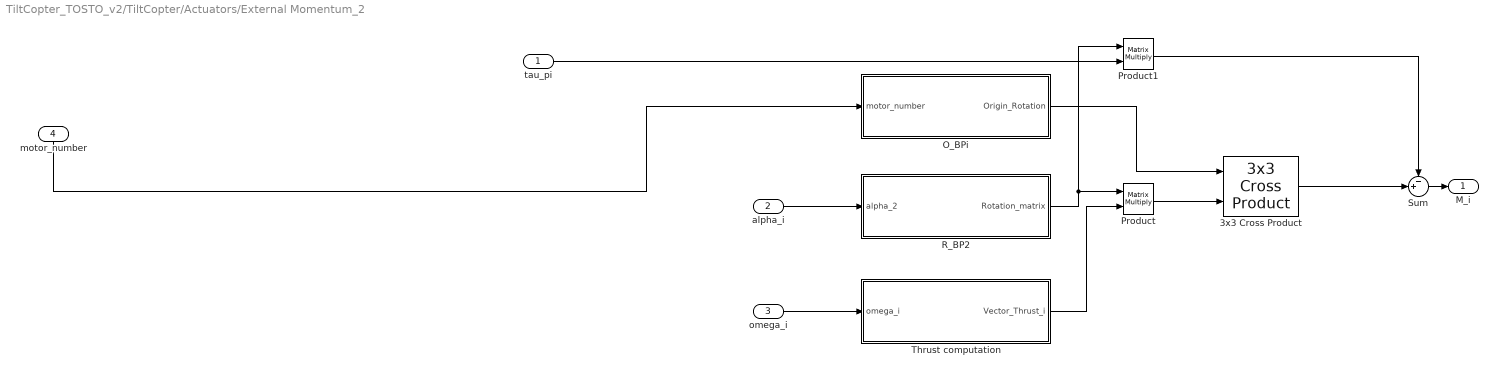
== system TiltCopter_TOSTO_v2/TiltCopter/Actuators/External Momentum_2 ==
  tau_pi : Inport
  alpha_i : Inport  Port=2
  omega_i : Inport  Port=3
  motor_number : Inport  Port=4
  3x3 Cross Product : aerolibutil/3x3 Cross Product
  O_BPi : MATLAB Function  TreatAsAtomicUnit=on
  Product : Product  Multiplication=Matrix(*)
  Product1 : Product  Multiplication=Matrix(*)
  R_BP2 : MATLAB Function  TreatAsAtomicUnit=on
  Sum : Sum  Inputs=-+|
  Thrust computation : Subsystem
  M_i : Outport
  wires:
  Sum/1 -> M_i/1
  R_BP2/1(Rotation_matrix) -> Product1/1, Product/1
  alpha_i/1 -> R_BP2/1(alpha_2)
  Product/1 -> 3x3 Cross Product/2
  tau_pi/1 -> Product1/2
  motor_number/1 -> O_BPi/1(motor_number)
  omega_i/1 -> Thrust computation/1(omega_i)
  Thrust computation/1(Vector_Thrust_i) -> Product/2
  3x3 Cross Product/1 -> Sum/2
  Product1/1 -> Sum/1
  O_BPi/1(Origin_Rotation) -> 3x3 Cross Product/1

== system TiltCopter_TOSTO_v2/TiltCopter/Actuators/External Momentum_3 ==
  tau_pi : Inport
  alpha_i : Inport  Port=2
  omega_i : Inport  Port=3
  motor_number : Inport  Port=4
  3x3 Cross Product : aerolibutil/3x3 Cross Product
  O_BPi : MATLAB Function  TreatAsAtomicUnit=on
  Product : Product  Multiplication=Matrix(*)
  Product1 : Product  Multiplication=Matrix(*)
  R_BP3 : MATLAB Function  TreatAsAtomicUnit=on
  Sum : Sum  Inputs=-+|
  Thrust computation : Subsystem
  M_i : Outport
  wires:
  Sum/1 -> M_i/1
  R_BP3/1(Rotation_matrix) -> Product1/1, Product/1
  alpha_i/1 -> R_BP3/1(alpha_3)
  Product/1 -> 3x3 Cross Product/2
  tau_pi/1 -> Product1/2
  motor_number/1 -> O_BPi/1(motor_number)
  omega_i/1 -> Thrust computation/1(omega_i)
  Thrust computation/1(Vector_Thrust_i) -> Product/2
  3x3 Cross Product/1 -> Sum/2
  Product1/1 -> Sum/1
  O_BPi/1(Origin_Rotation) -> 3x3 Cross Product/1

== system TiltCopter_TOSTO_v2/TiltCopter/Actuators/External Momentum_4 ==
  tau_pi : Inport
  alpha_i : Inport  Port=2
  omega_i : Inport  Port=3
  motor_number : Inport  Port=4
  3x3 Cross Product : aerolibutil/3x3 Cross Product
  O_BPi : MATLAB Function  TreatAsAtomicUnit=on
  Product : Product  Multiplication=Matrix(*)
  Product1 : Product  Multiplication=Matrix(*)
  R_BP4 : MATLAB Function  TreatAsAtomicUnit=on
  Sum : Sum  Inputs=-+|
  Thrust computation : Subsystem
  M_i : Outport
  wires:
  Sum/1 -> M_i/1
  R_BP4/1(Rotation_matrix) -> Product1/1, Product/1
  alpha_i/1 -> R_BP4/1(alpha_4)
  Product/1 -> 3x3 Cross Product/2
  tau_pi/1 -> Product1/2
  motor_number/1 -> O_BPi/1(motor_number)
  omega_i/1 -> Thrust computation/1(omega_i)
  Thrust computation/1(Vector_Thrust_i) -> Product/2
  3x3 Cross Product/1 -> Sum/2
  Product1/1 -> Sum/1
  O_BPi/1(Origin_Rotation) -> 3x3 Cross Product/1

== system TiltCopter_TOSTO_v2/TiltCopter/Actuators/Servo_Motor 1 ==
  Pulse_1 [ms] : Inport
  "Angle [rad] -> Pulse [ms]" : Subsystem
  Derivative : Derivative
  Derivative1 : Derivative
  Gain : Gain  Gain=ServoMotor_Gain
  Transfer Fcn : TransferFcn  Denominator=[B3 B2 B1 B0]
  alpha_1 [rad] : Outport
  dalpha_1 : Outport  Port=2
  ddalpha_1 : Outport  Port=3
  wires:
  Gain/1 -> Derivative/1, alpha_1 [rad]/1
  Transfer Fcn/1 -> Gain/1
  "Angle [rad] -> Pulse [ms]"/1(Angle [rad]) -> Transfer Fcn/1
  Pulse_1 [ms]/1 -> "Angle [rad] -> Pulse [ms]"/1(Pulse [ms])
  Derivative/1 -> dalpha_1/1, Derivative1/1
  Derivative1/1 -> ddalpha_1/1

== system TiltCopter_TOSTO_v2/TiltCopter/Actuators/Servo_Motor 2 ==
  Pulse_2 [ms] : Inport
  "Angle [rad] -> Pulse [ms]" : Subsystem
  Derivative : Derivative
  Derivative1 : Derivative
  Gain : Gain  Gain=ServoMotor_Gain
  Transfer Fcn : TransferFcn  Denominator=[B3 B2 B1 B0]
  alpha_2 [rad] : Outport
  dalpha_2 : Outport  Port=2
  ddalpha_2 : Outport  Port=3
  wires:
  Gain/1 -> Derivative/1, alpha_2 [rad]/1
  Transfer Fcn/1 -> Gain/1
  "Angle [rad] -> Pulse [ms]"/1(Angle [rad]) -> Transfer Fcn/1
  Pulse_2 [ms]/1 -> "Angle [rad] -> Pulse [ms]"/1(Pulse [ms])
  Derivative/1 -> dalpha_2/1, Derivative1/1
  Derivative1/1 -> ddalpha_2/1

== system TiltCopter_TOSTO_v2/TiltCopter/Actuators/Servo_Motor 3 ==
  Pulse_3 [ms] : Inport
  "Angle [rad] -> Pulse [ms]" : Subsystem
  Derivative : Derivative
  Derivative1 : Derivative
  Gain : Gain  Gain=ServoMotor_Gain
  Transfer Fcn : TransferFcn  Denominator=[B3 B2 B1 B0]
  alpha_3 [rad] : Outport
  dalpha_3 : Outport  Port=2
  ddalpha_3 : Outport  Port=3
  wires:
  Gain/1 -> Derivative/1, alpha_3 [rad]/1
  Transfer Fcn/1 -> Gain/1
  "Angle [rad] -> Pulse [ms]"/1(Angle [rad]) -> Transfer Fcn/1
  Pulse_3 [ms]/1 -> "Angle [rad] -> Pulse [ms]"/1(Pulse [ms])
  Derivative/1 -> dalpha_3/1, Derivative1/1
  Derivative1/1 -> ddalpha_3/1

== system TiltCopter_TOSTO_v2/TiltCopter/Actuators/Servo_Motor 4 ==
  Pulse_4 [ms] : Inport
  "Angle [rad] -> Pulse [ms]" : Subsystem
  Derivative : Derivative
  Derivative1 : Derivative
  Gain : Gain  Gain=ServoMotor_Gain
  Transfer Fcn : TransferFcn  Denominator=[B3 B2 B1 B0]
  alpha_4 [rad] : Outport
  dalpha_4 : Outport  Port=2
  ddalpha_4 : Outport  Port=3
  wires:
  Gain/1 -> Derivative/1, alpha_4 [rad]/1
  Transfer Fcn/1 -> Gain/1
  "Angle [rad] -> Pulse [ms]"/1(Angle [rad]) -> Transfer Fcn/1
  Pulse_4 [ms]/1 -> "Angle [rad] -> Pulse [ms]"/1(Pulse [ms])
  Derivative1/1 -> ddalpha_4/1
  Derivative/1 -> Derivative1/1, dalpha_4/1

== system TiltCopter_TOSTO_v2/TiltCopter/Actuators/Traslational Force_1 ==
  alpha_i : Inport
  omega_i : Inport  Port=2
  Product : Product  Multiplication=Matrix(*)
  R_BP1 : MATLAB Function  TreatAsAtomicUnit=on
  Thrust computation : Subsystem
  F_i : Outport
  wires:
  Thrust computation/1(Vector_Thrust_i) -> Product/2
  Product/1 -> F_i/1
  omega_i/1 -> Thrust computation/1(omega_i)
  R_BP1/1(Rotation_matrix) -> Product/1
  alpha_i/1 -> R_BP1/1(alpha_1)

== system TiltCopter_TOSTO_v2/TiltCopter/Actuators/Traslational Force_2 ==
  alpha_i : Inport
  omega_i : Inport  Port=2
  Product : Product  Multiplication=Matrix(*)
  R_BP2 : MATLAB Function  TreatAsAtomicUnit=on
  Thrust computation : Subsystem
  F_i : Outport
  wires:
  Thrust computation/1(Vector_Thrust_i) -> Product/2
  Product/1 -> F_i/1
  omega_i/1 -> Thrust computation/1(omega_i)
  R_BP2/1(Rotation_matrix) -> Product/1
  alpha_i/1 -> R_BP2/1(alpha_2)

== system TiltCopter_TOSTO_v2/TiltCopter/Actuators/Traslational Force_3 ==
  alpha_i : Inport
  omega_i : Inport  Port=2
  Product : Product  Multiplication=Matrix(*)
  R_BP3 : MATLAB Function  TreatAsAtomicUnit=on
  Thrust computation : Subsystem
  F_i : Outport
  wires:
  Thrust computation/1(Vector_Thrust_i) -> Product/2
  Product/1 -> F_i/1
  omega_i/1 -> Thrust computation/1(omega_i)
  R_BP3/1(Rotation_matrix) -> Product/1
  alpha_i/1 -> R_BP3/1(alpha_3)

== system TiltCopter_TOSTO_v2/TiltCopter/Actuators/Traslational Force_4 ==
  alpha_i : Inport
  omega_i : Inport  Port=2
  Product : Product  Multiplication=Matrix(*)
  R_BP4 : MATLAB Function  TreatAsAtomicUnit=on
  Thrust computation : Subsystem
  F_i : Outport
  wires:
  Thrust computation/1(Vector_Thrust_i) -> Product/2
  Product/1 -> F_i/1
  omega_i/1 -> Thrust computation/1(omega_i)
  R_BP4/1(Rotation_matrix) -> Product/1
  alpha_i/1 -> R_BP4/1(alpha_4)

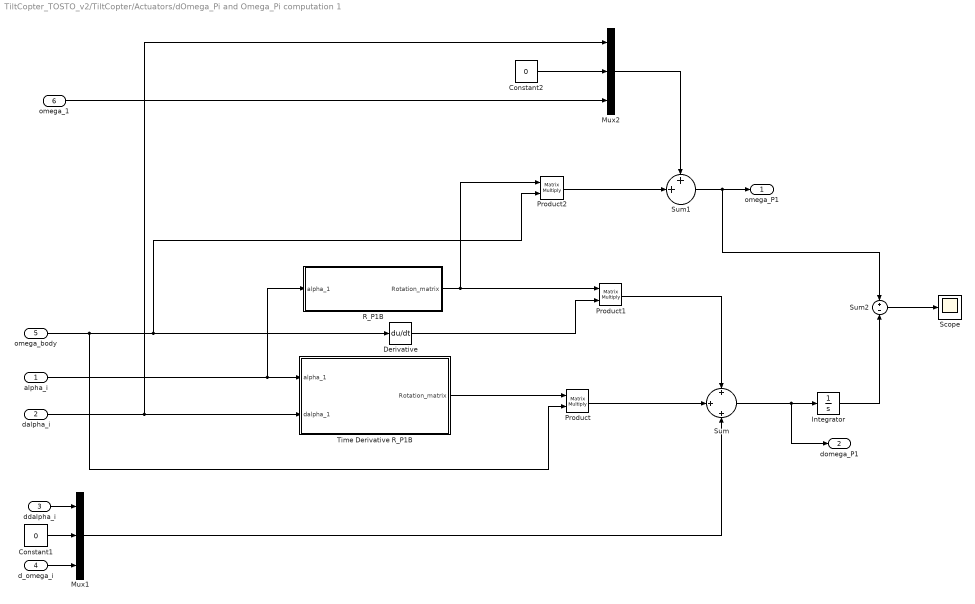
== system TiltCopter_TOSTO_v2/TiltCopter/Actuators/dOmega_Pi and Omega_Pi computation 1 ==
  alpha_i : Inport
  dalpha_i : Inport  Port=2
  ddalpha_i : Inport  Port=3
  d_omega_i : Inport  Port=4
  omega_body : Inport  Port=5
  omega_1 : Inport  Port=6
  Constant1 : Constant  Value=0
  Constant2 : Constant  Value=0
  Derivative : Derivative
  Integrator : Integrator
  Mux1 : Mux  Inputs=3
  Mux2 : Mux  Inputs=3
  Product : Product  Multiplication=Matrix(*)
  Product1 : Product  Multiplication=Matrix(*)
  Product2 : Product  Multiplication=Matrix(*)
  R_P1B : MATLAB Function  TreatAsAtomicUnit=on
  Scope : Scope
      settings: ShowLegends=on  SaveName=ScopeData29
  Sum : Sum  Inputs=+|+|+
  Sum1 : Sum  Inputs=++|
  Sum2 : Sum  Inputs=+-
  Time Derivative R_P1B : MATLAB Function  TreatAsAtomicUnit=on
  omega_P1 : Outport
  domega_P1 : Outport  Port=2
  wires:
  Derivative/1 -> Product1/2
  Product/1 -> Sum/2
  Time Derivative R_P1B/1(Rotation_matrix) -> Product/1
  Constant1/1 -> Mux1/2
  omega_body/1 -> Product/2, Product2/2, Derivative/1
  dalpha_i/1 -> Mux2/1, Time Derivative R_P1B/2(dalpha_1)
  alpha_i/1 -> R_P1B/1(alpha_1), Time Derivative R_P1B/1(alpha_1)
  R_P1B/1(Rotation_matrix) -> Product2/1, Product1/1
  Sum/1 -> domega_P1/1, Integrator/1
  Product1/1 -> Sum/1
  Mux1/1 -> Sum/3
  ddalpha_i/1 -> Mux1/1
  Product2/1 -> Sum1/2
  Constant2/1 -> Mux2/2
  Mux2/1 -> Sum1/1
  Sum1/1 -> Sum2/1, omega_P1/1
  omega_1/1 -> Mux2/3
  d_omega_i/1 -> Mux1/3
  Integrator/1 -> Sum2/2
  Sum2/1 -> Scope/1

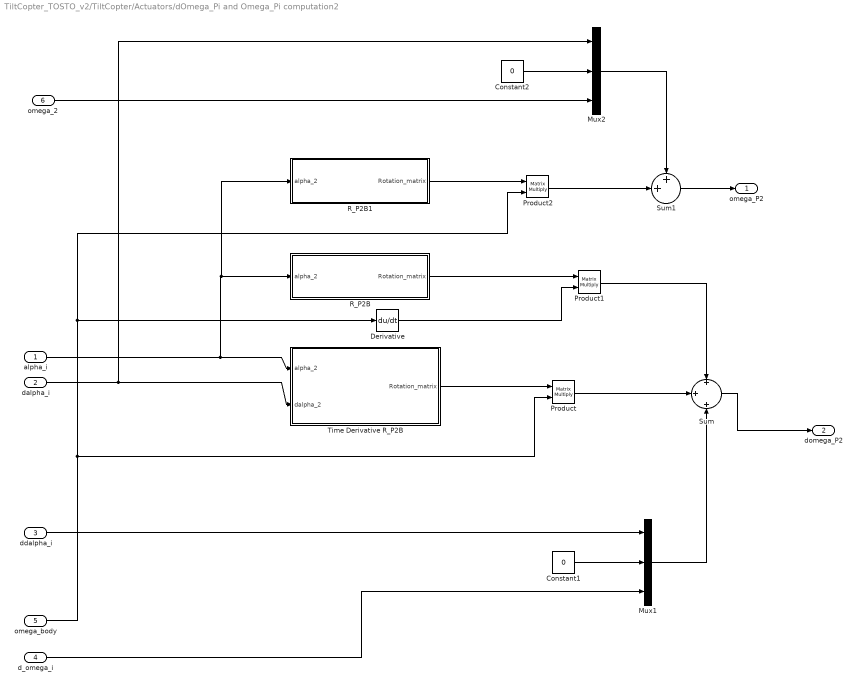
== system TiltCopter_TOSTO_v2/TiltCopter/Actuators/dOmega_Pi and Omega_Pi computation2 ==
  alpha_i : Inport
  dalpha_i : Inport  Port=2
  ddalpha_i : Inport  Port=3
  d_omega_i : Inport  Port=4
  omega_body : Inport  Port=5
  omega_2 : Inport  Port=6
  Constant1 : Constant  Value=0
  Constant2 : Constant  Value=0
  Derivative : Derivative
  Mux1 : Mux  Inputs=3
  Mux2 : Mux  Inputs=3
  Product : Product  Multiplication=Matrix(*)
  Product1 : Product  Multiplication=Matrix(*)
  Product2 : Product  Multiplication=Matrix(*)
  R_P2B : MATLAB Function  TreatAsAtomicUnit=on
  R_P2B1 : MATLAB Function  TreatAsAtomicUnit=on
  Sum : Sum  Inputs=+|+|+
  Sum1 : Sum  Inputs=++|
  Time Derivative R_P2B : MATLAB Function  TreatAsAtomicUnit=on
  omega_P2 : Outport
  domega_P2 : Outport  Port=2
  wires:
  Derivative/1 -> Product1/2
  Product/1 -> Sum/2
  Time Derivative R_P2B/1(Rotation_matrix) -> Product/1
  Constant1/1 -> Mux1/2
  omega_body/1 -> Product/2, Product2/2, Derivative/1
  dalpha_i/1 -> Mux2/1, Time Derivative R_P2B/2(dalpha_2)
  alpha_i/1 -> R_P2B1/1(alpha_2), R_P2B/1(alpha_2), Time Derivative R_P2B/1(alpha_2)
  Sum/1 -> domega_P2/1
  Product1/1 -> Sum/1
  Mux1/1 -> Sum/3
  ddalpha_i/1 -> Mux1/1
  R_P2B/1(Rotation_matrix) -> Product1/1
  R_P2B1/1(Rotation_matrix) -> Product2/1
  Product2/1 -> Sum1/2
  Constant2/1 -> Mux2/2
  Mux2/1 -> Sum1/1
  Sum1/1 -> omega_P2/1
  d_omega_i/1 -> Mux1/3
  omega_2/1 -> Mux2/3

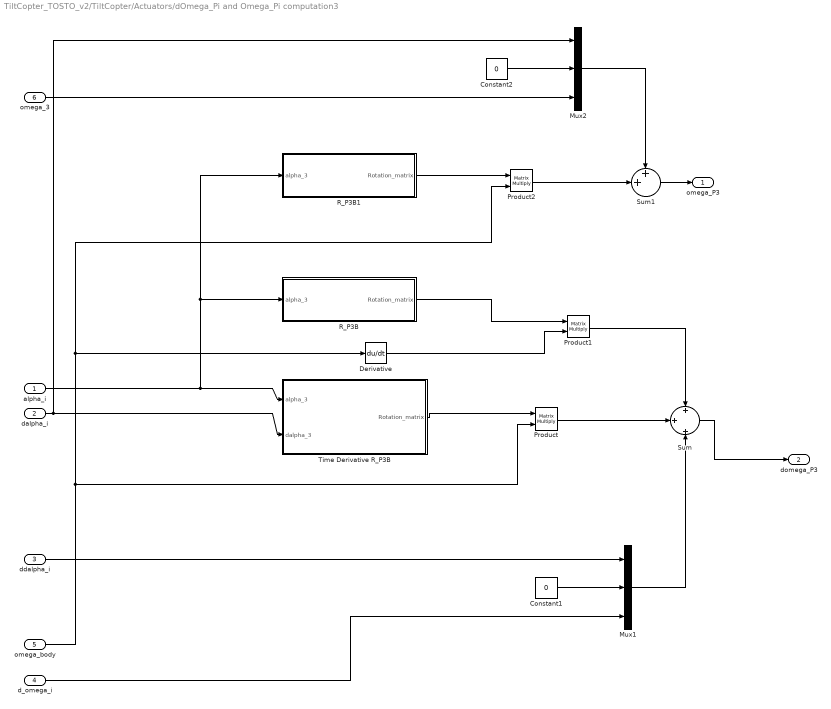
== system TiltCopter_TOSTO_v2/TiltCopter/Actuators/dOmega_Pi and Omega_Pi computation3 ==
  alpha_i : Inport
  dalpha_i : Inport  Port=2
  ddalpha_i : Inport  Port=3
  d_omega_i : Inport  Port=4
  omega_body : Inport  Port=5
  omega_3 : Inport  Port=6
  Constant1 : Constant  Value=0
  Constant2 : Constant  Value=0
  Derivative : Derivative
  Mux1 : Mux  Inputs=3
  Mux2 : Mux  Inputs=3
  Product : Product  Multiplication=Matrix(*)
  Product1 : Product  Multiplication=Matrix(*)
  Product2 : Product  Multiplication=Matrix(*)
  R_P3B : MATLAB Function  TreatAsAtomicUnit=on
  R_P3B1 : MATLAB Function  TreatAsAtomicUnit=on
  Sum : Sum  Inputs=+|+|+
  Sum1 : Sum  Inputs=++|
  Time Derivative R_P3B : MATLAB Function  TreatAsAtomicUnit=on
  omega_P3 : Outport
  domega_P3 : Outport  Port=2
  wires:
  Derivative/1 -> Product1/2
  Product/1 -> Sum/2
  Time Derivative R_P3B/1(Rotation_matrix) -> Product/1
  Constant1/1 -> Mux1/2
  omega_body/1 -> Product/2, Product2/2, Derivative/1
  alpha_i/1 -> R_P3B1/1(alpha_3), R_P3B/1(alpha_3), Time Derivative R_P3B/1(alpha_3)
  Sum/1 -> domega_P3/1
  Product1/1 -> Sum/1
  Mux1/1 -> Sum/3
  ddalpha_i/1 -> Mux1/1
  R_P3B/1(Rotation_matrix) -> Product1/1
  R_P3B1/1(Rotation_matrix) -> Product2/1
  Product2/1 -> Sum1/2
  Constant2/1 -> Mux2/2
  Mux2/1 -> Sum1/1
  dalpha_i/1 -> Mux2/1, Time Derivative R_P3B/2(dalpha_3)
  Sum1/1 -> omega_P3/1
  d_omega_i/1 -> Mux1/3
  omega_3/1 -> Mux2/3

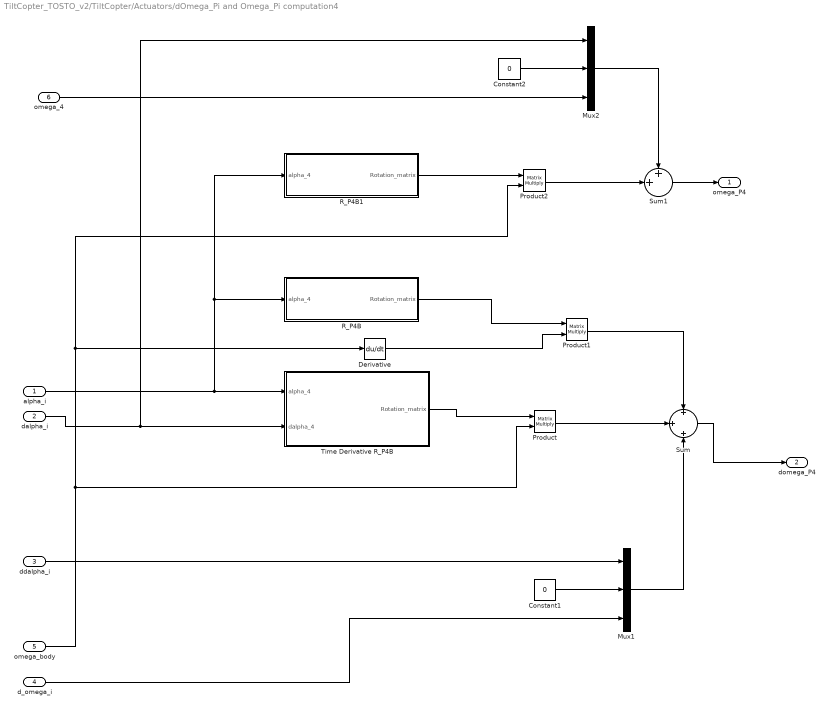
== system TiltCopter_TOSTO_v2/TiltCopter/Actuators/dOmega_Pi and Omega_Pi computation4 ==
  alpha_i : Inport
  dalpha_i : Inport  Port=2
  ddalpha_i : Inport  Port=3
  d_omega_i : Inport  Port=4
  omega_body : Inport  Port=5
  omega_4 : Inport  Port=6
  Constant1 : Constant  Value=0
  Constant2 : Constant  Value=0
  Derivative : Derivative
  Mux1 : Mux  Inputs=3
  Mux2 : Mux  Inputs=3
  Product : Product  Multiplication=Matrix(*)
  Product1 : Product  Multiplication=Matrix(*)
  Product2 : Product  Multiplication=Matrix(*)
  R_P4B : MATLAB Function  TreatAsAtomicUnit=on
  R_P4B1 : MATLAB Function  TreatAsAtomicUnit=on
  Sum : Sum  Inputs=+|+|+
  Sum1 : Sum  Inputs=++|
  Time Derivative R_P4B : MATLAB Function  TreatAsAtomicUnit=on
  omega_P4 : Outport
  domega_P4 : Outport  Port=2
  wires:
  Derivative/1 -> Product1/2
  Product/1 -> Sum/2
  Time Derivative R_P4B/1(Rotation_matrix) -> Product/1
  Constant1/1 -> Mux1/2
  omega_body/1 -> Product/2, Product2/2, Derivative/1
  dalpha_i/1 -> Mux2/1, Time Derivative R_P4B/2(dalpha_4)
  alpha_i/1 -> R_P4B1/1(alpha_4), R_P4B/1(alpha_4), Time Derivative R_P4B/1(alpha_4)
  Sum/1 -> domega_P4/1
  Product1/1 -> Sum/1
  Mux1/1 -> Sum/3
  ddalpha_i/1 -> Mux1/1
  R_P4B/1(Rotation_matrix) -> Product1/1
  Product2/1 -> Sum1/2
  Constant2/1 -> Mux2/2
  Mux2/1 -> Sum1/1
  R_P4B1/1(Rotation_matrix) -> Product2/1
  Sum1/1 -> omega_P4/1
  omega_4/1 -> Mux2/3
  d_omega_i/1 -> Mux1/3

== system TiltCopter_TOSTO_v2/TiltCopter/Actuators/tau_p1 computation ==
  omega_P1 : Inport
  domega_P1 : Inport  Port=2
  omega_i : Inport  Port=3
  3x3 Cross Product : aerolibutil/3x3 Cross Product
  Constant : Constant  Value=I_Pi
  Drag torque computation : Subsystem
  Gain : Gain  Gain=[1;1;-1]
  Product : Product  Multiplication=Matrix(*)
  Product1 : Product  Multiplication=Matrix(*)
  Sum : Sum  Inputs=+|+|-
  tau_P1 : Outport
  wires:
  Constant/1 -> Product/1, Product1/1
  omega_P1/1 -> 3x3 Cross Product/1, Product1/2
  Product/1 -> Sum/2
  domega_P1/1 -> Product/2
  Product1/1 -> 3x3 Cross Product/2
  Sum/1 -> tau_P1/1
  3x3 Cross Product/1 -> Sum/1
  Drag torque computation/1(Vector_DragTorque_i) -> Gain/1
  omega_i/1 -> Drag torque computation/1(omega_P1_z)
  Gain/1 -> Sum/3

== system TiltCopter_TOSTO_v2/TiltCopter/Actuators/tau_p2 computation ==
  omega_P2 : Inport
  domega_P2 : Inport  Port=2
  omega_i : Inport  Port=3
  3x3 Cross Product : aerolibutil/3x3 Cross Product
  Constant : Constant  Value=I_Pi
  Drag torque computation : Subsystem
  Gain : Gain  Gain=[1;1;-1]
  Product : Product  Multiplication=Matrix(*)
  Product1 : Product  Multiplication=Matrix(*)
  Sum : Sum  Inputs=+|+|-
  tau_P2 : Outport
  wires:
  3x3 Cross Product/1 -> Sum/1
  Sum/1 -> tau_P2/1
  Product1/1 -> 3x3 Cross Product/2
  domega_P2/1 -> Product/2
  Product/1 -> Sum/2
  omega_P2/1 -> Product1/2, 3x3 Cross Product/1
  Constant/1 -> Product/1, Product1/1
  Drag torque computation/1(Vector_DragTorque_i) -> Gain/1
  omega_i/1 -> Drag torque computation/1(omega_P2)
  Gain/1 -> Sum/3

== system TiltCopter_TOSTO_v2/TiltCopter/Actuators/tau_p3 computation1 ==
  omega_P3 : Inport
  domega_P3 : Inport  Port=2
  omega_i : Inport  Port=3
  3x3 Cross Product : aerolibutil/3x3 Cross Product
  Constant : Constant  Value=I_Pi
  Drag torque computation : Subsystem
  Gain : Gain  Gain=[1;1;-1]
  Product : Product  Multiplication=Matrix(*)
  Product1 : Product  Multiplication=Matrix(*)
  Sum : Sum  Inputs=+|+|-
  tau_P3 : Outport
  wires:
  Constant/1 -> Product1/1, Product/1
  omega_P3/1 -> 3x3 Cross Product/1, Product1/2
  Product/1 -> Sum/2
  domega_P3/1 -> Product/2
  Product1/1 -> 3x3 Cross Product/2
  Sum/1 -> tau_P3/1
  3x3 Cross Product/1 -> Sum/1
  Drag torque computation/1(Vector_DragTorque_i) -> Gain/1
  omega_i/1 -> Drag torque computation/1(omega_P3)
  Gain/1 -> Sum/3

== system TiltCopter_TOSTO_v2/TiltCopter/Actuators/tau_p4 computation2 ==
  omega_P4 : Inport
  domega_P4 : Inport  Port=2
  omega_i : Inport  Port=3
  3x3 Cross Product : aerolibutil/3x3 Cross Product
  Constant : Constant  Value=I_Pi
  Drag torque computation : Subsystem
  Gain : Gain  Gain=[1;1;-1]
  Product : Product  Multiplication=Matrix(*)
  Product1 : Product  Multiplication=Matrix(*)
  Sum : Sum  Inputs=+|+|-
  tau_P4 : Outport
  wires:
  3x3 Cross Product/1 -> Sum/1
  Sum/1 -> tau_P4/1
  Product1/1 -> 3x3 Cross Product/2
  domega_P4/1 -> Product/2
  Product/1 -> Sum/2
  omega_P4/1 -> Product1/2, 3x3 Cross Product/1
  Constant/1 -> Product/1, Product1/1
  Drag torque computation/1(Vector_DragTorque_i) -> Gain/1
  omega_i/1 -> Drag torque computation/1(omega_P4)
  Gain/1 -> Sum/3
